simulink model "BergmanModel"  (R2021a)
settings: Solver=VariableStepAuto  StartTime=0.0  StopTime=1000  RelTol=1e-3
model workspace (MAT data in the model file):
  U1 = 10
  u2 = 100
settings Model: Creator=marti  LastModifiedBy=marti
settings SolverCC: AlgebraicLoopSolver=TrustRegion
settings DataIOCC: ReturnWorkspaceOutputs=off
settings DebuggingCC: SFMachineParentedDataDiag=warning  ArithmeticOperatorsInVariantConditions=warning
settings SFSimCC: CustomCodeUndefinedFunction=UseInterfaceOnly

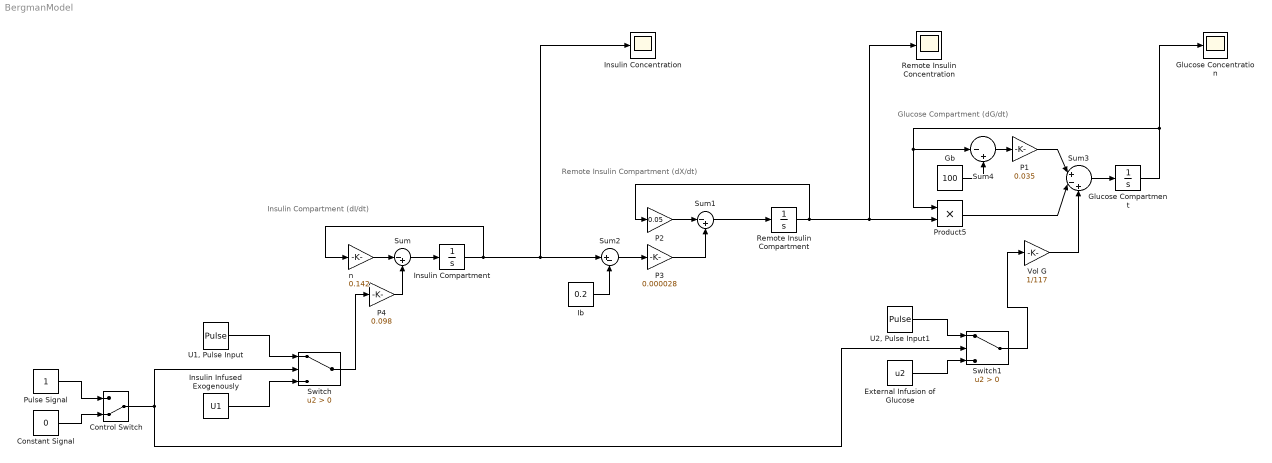
== system BergmanModel ==
  note: Insulin Compartment (dI/dt)
  note: Glucose Compartment (dG/dt)
  note: Remote Insulin Compartment (dX/dt)
  Constant Signal : Constant  Value=0
  Control Switch : ManualSwitch  CurrentSetting=0
  External Infusion of Glucose : Constant  Value=u2
  Gb : Constant  Value=100
  Glucose Compartment : Integrator  InitialCondition=100
  Glucose Concentration : Scope
  Ib : Constant  Value=0.2
  Insulin Compartment : Integrator
  Insulin Concentration : Scope
  Insulin Infused Exogenously : Constant  Value=U1  OutMin=0  OutMax=1000
  P1 : Gain  Gain=0.035
  P2 : Gain  Gain=0.05
  P3 : Gain  Gain=0.000028
  P4 : Gain  Gain=0.098
  Product5 : Product
  Pulse Signal : Constant
  Remote Insulin Compartment : Integrator
  Remote Insulin Concentration : Scope
  Sum : Sum  Inputs=|-+
  Sum1 : Sum  Inputs=|-+
  Sum2 : Sum  Inputs=|+-
  Sum3 : Sum  Inputs=|+-+
  Sum4 : Sum  Inputs=|-+
  Switch : Switch  Criteria=u2 > Threshold
  Switch1 : Switch  Criteria=u2 > Threshold
  "U1, Pulse Input" : DiscretePulseGenerator  PulseType=Time based  Amplitude=0  Period=1000  PulseWidth=.5  PhaseDelay=20
  "U2, Pulse Input1" : DiscretePulseGenerator  PulseType=Time based  Amplitude=100  Period=1000  PulseWidth=.5  PhaseDelay=10
  Vol G : Gain  Gain=1/117
  n : Gain  Gain=0.142
  wires:
  Remote Insulin Compartment/1 -> P2/1, Remote Insulin Concentration/1, Product5/2
  Insulin Compartment/1 -> n/1, Insulin Concentration/1, Sum2/1
  Product5/1 -> Sum3/2
  n/1 -> Sum/1
  P3/1 -> Sum1/2
  Sum1/1 -> Remote Insulin Compartment/1
  Gb/1 -> Sum4/2
  Sum/1 -> Insulin Compartment/1
  P2/1 -> Sum1/1
  Sum3/1 -> Glucose Compartment/1
  P1/1 -> Sum3/1
  Sum4/1 -> P1/1
  P4/1 -> Sum/2
  Glucose Compartment/1 -> Product5/1, Sum4/1, Glucose Concentration/1
  Ib/1 -> Sum2/2
  Sum2/1 -> P3/1
  Vol G/1 -> Sum3/3
  Control Switch/1 -> Switch/2, Switch1/2
  Pulse Signal/1 -> Control Switch/1
  Constant Signal/1 -> Control Switch/2
  External Infusion of Glucose/1 -> Switch1/3
  "U2, Pulse Input1"/1 -> Switch1/1
  Switch1/1 -> Vol G/1
  Switch/1 -> P4/1
  "U1, Pulse Input"/1 -> Switch/1
  Insulin Infused Exogenously/1 -> Switch/3
